simulink model "model"  (R2016a)
settings: Solver=VariableStepAuto  StartTime=0.0  StopTime=30  FixedStep=0.001  RelTol=1e-3
InitFcn:
  | InitModel;
values from neighbouring files (symbols this model uses):
  d = 100    [InitModel.m]    (also in RobotConstants.mat = 1000)
  k = 1900    [RobotConstants.mat]
  l0 = 0.16    [RobotConstants.mat]
  ls = 0.17    [RobotConstants.mat]
  m_lower = 0.5    [RobotConstants.mat]
  m_upper = 1    [RobotConstants.mat]
  n = ceil(length(q)/3)    [C.m]    (also in InitModel.m = 1; M.m; N.m; Q.m)
settings Model: Creator=Florian  LastModifiedBy=Florian
settings DataIOCC: ExternalInput=[l0]

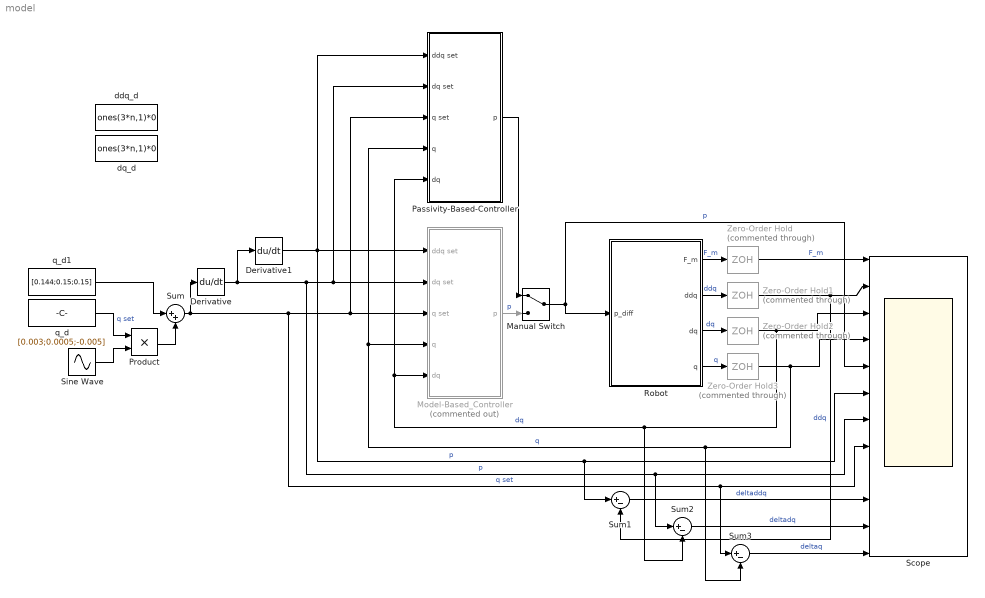
== system model ==
  Derivative : Derivative
  Derivative1 : Derivative
  Manual Switch : ManualSwitch
  Model-Based_Controller : Subsystem  Commented=on
  Passivity-Based-Controller : Subsystem
  Product : Product
  Robot : Subsystem
      mask Display: image('C:\Users\Florian\Documents\Uni\IDP\DVD\Pictures\contibot1seg.JPG');
  Scope : Scope  NumInputPorts=12
  Sine Wave : Sin  Amplitude=0.5  Bias=0.5  Phase=pi/2  SampleTime=0
  Sum : Sum  Inputs=|++
  Sum1 : Sum  Inputs=|+-
  Sum2 : Sum  Inputs=|+-
  Sum3 : Sum  Inputs=|+-
  Zero-Order Hold{,1..3} (4 alike) : ZeroOrderHold  Commented=through  SampleTime=0.01
  ddq_d : Constant  Value=ones(3*n,1)*0  SampleTime=0.01
  dq_d : Constant  Value=ones(3*n,1)*0  SampleTime=0.01
  q_d : Constant  Value=[0.003;0.0005;-0.005]  SampleTime=0.01
  q_d1 : Constant  Value=[0.144;0.15;0.15]  SampleTime=0.01
  wires:
  Robot/1(F_m) -> Zero-Order Hold/1  "F_m"
  Robot/2(ddq) -> Zero-Order Hold1/1  "ddq"
  Robot/3(dq) -> Zero-Order Hold2/1  "dq"
  Robot/4(q) -> Zero-Order Hold3/1  "q"
  Sum/1 -> Derivative/1, Sum3/1, Scope/8, Passivity-Based-Controller/3(q set), Model-Based_Controller/3(q set)  "q set"
  Zero-Order Hold/1 -> Scope/1  "F_m"
  Zero-Order Hold1/1 -> Sum1/2, Scope/2  "ddq"
  Zero-Order Hold2/1 -> Model-Based_Controller/5(dq), Passivity-Based-Controller/5(dq), Sum2/2, Scope/3  "dq"
  Zero-Order Hold3/1 -> Passivity-Based-Controller/4(q), Model-Based_Controller/4(q), Sum3/2, Scope/4  "q"
  Derivative/1 -> Passivity-Based-Controller/2(dq set), Model-Based_Controller/2(dq set), Sum2/1, Scope/7, Derivative1/1  "p"
  Derivative1/1 -> Passivity-Based-Controller/1(ddq set), Model-Based_Controller/1(ddq set), Sum1/1, Scope/6  "p"
  Manual Switch/1 -> Robot/1(p_diff), Scope/5  "p"
  Model-Based_Controller/1(p) -> Manual Switch/2  "p"
  Passivity-Based-Controller/1(p) -> Manual Switch/1
  q_d/1 -> Product/1  "q set"
  Sine Wave/1 -> Product/2
  Product/1 -> Sum/2
  q_d1/1 -> Sum/1
  Sum3/1 -> Scope/12  "deltaq"
  Sum2/1 -> Scope/11  "deltadq"
  Sum1/1 -> Scope/10  "deltaddq"

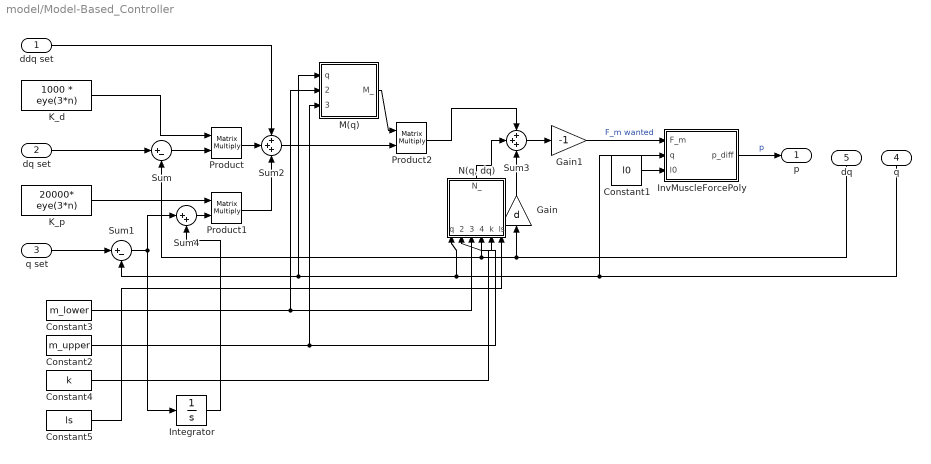
== system model/Model-Based_Controller ==
  ddq set : Inport
  dq set : Inport  Port=2
  q set : Inport  Port=3
  q : Inport  Port=4
  dq : Inport  Port=5
  Constant1 : Constant  Value=l0  SampleTime=0.01
  Constant2 : Constant  Value=m_upper
  Constant3 : Constant  Value=m_lower
  Constant4 : Constant  Value=k
  Constant5 : Constant  Value=ls
  Gain : Gain  Gain=d
  Gain1 : Gain  Gain=-1
  Integrator : Integrator  InitialCondition=zeros(3*n,1)
  InvMuscleForcePoly : MATLAB Function  TreatAsAtomicUnit=on
  K_d : Constant  Value=1000 * eye(3*n)  SampleTime=0.01
  K_p : Constant  Value=20000* eye(3*n)  SampleTime=0.01
  M(q) : MATLAB Function  TreatAsAtomicUnit=on
  "N(q, dq)" : MATLAB Function  TreatAsAtomicUnit=on
  Product : Product  Multiplication=Matrix(*)
  Product1 : Product  Multiplication=Matrix(*)
  Product2 : Product  Multiplication=Matrix(*)
  Sum : Sum  Inputs=|+-
  Sum1 : Sum  Inputs=|+-
  Sum2 : Sum  Inputs=+++
  Sum3 : Sum  Inputs=+++
  Sum4 : Sum  Inputs=|++
  p : Outport
  wires:
  Sum/1 -> Product/2
  M(q)/1(M_) -> Product2/1
  Sum2/1 -> Product2/2
  "N(q, dq)"/1(N_) -> Sum3/2
  K_p/1 -> Product1/1
  Gain/1 -> Sum3/3
  Sum1/1 -> Sum4/1, Integrator/1
  Product1/1 -> Sum2/3
  Product2/1 -> Sum3/1
  Product/1 -> Sum2/2
  Sum3/1 -> Gain1/1
  K_d/1 -> Product/1
  Constant1/1 -> InvMuscleForcePoly/3(l0)
  Gain1/1 -> InvMuscleForcePoly/1(F_m)  "F_m wanted"
  InvMuscleForcePoly/1(p_diff) -> p/1  "p"
  dq/1 -> Sum/2, "N(q, dq)"/2(dq), Gain/1
  q set/1 -> Sum1/1
  q/1 -> Sum1/2, M(q)/1(q), "N(q, dq)"/1(q), InvMuscleForcePoly/2(q)
  dq set/1 -> Sum/1
  ddq set/1 -> Sum2/1
  Constant3/1 -> M(q)/2(m_lower), "N(q, dq)"/3(m_lower)
  Constant2/1 -> M(q)/3(m_upper), "N(q, dq)"/4(m_upper)
  Constant4/1 -> "N(q, dq)"/5(k)
  Constant5/1 -> "N(q, dq)"/6(ls)
  Integrator/1 -> Sum4/2
  Sum4/1 -> Product1/2

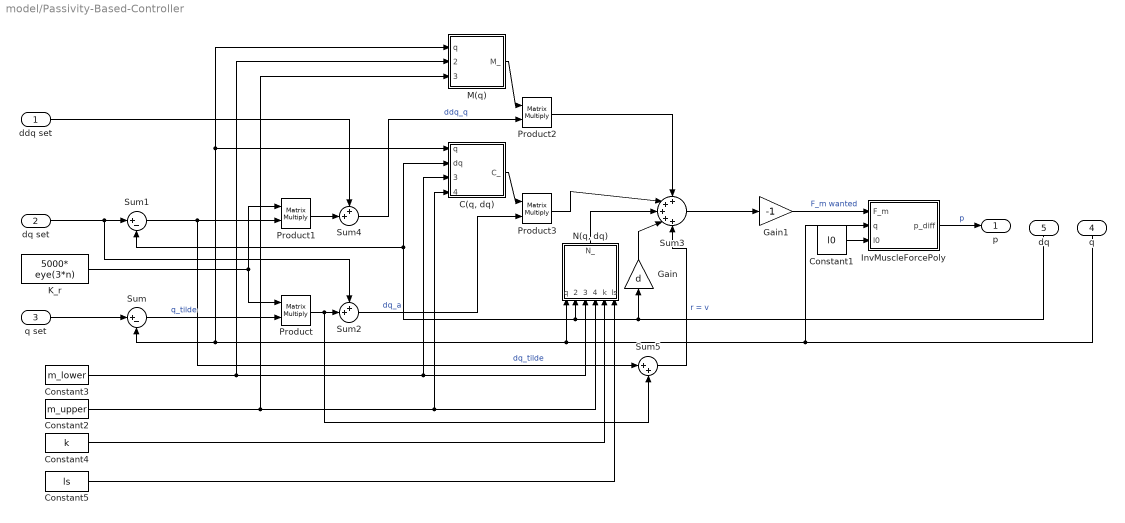
== system model/Passivity-Based-Controller ==
  ddq set : Inport
  dq set : Inport  Port=2
  q set : Inport  Port=3
  q : Inport  Port=4
  dq : Inport  Port=5
  "C(q, dq)" : MATLAB Function  TreatAsAtomicUnit=on
  Constant1 : Constant  Value=l0  SampleTime=0.01
  Constant2 : Constant  Value=m_upper
  Constant3 : Constant  Value=m_lower
  Constant4 : Constant  Value=k
  Constant5 : Constant  Value=ls
  Gain : Gain  Gain=d
  Gain1 : Gain  Gain=-1
  InvMuscleForcePoly : MATLAB Function  TreatAsAtomicUnit=on
  K_r : Constant  Value=5000* eye(3*n)  SampleTime=0.01
  M(q) : MATLAB Function  TreatAsAtomicUnit=on
  "N(q, dq)" : MATLAB Function  TreatAsAtomicUnit=on
  Product{,1..3} (4 alike) : Product  Multiplication=Matrix(*)
  Sum : Sum  Inputs=|+-
  Sum1 : Sum  Inputs=|+-
  Sum2 : Sum  Inputs=++|
  Sum3 : Sum  Inputs=+++++
  Sum4 : Sum  Inputs=++|
  Sum5 : Sum  Inputs=|++
  p : Outport
  wires:
  M(q)/1(M_) -> Product2/1
  "N(q, dq)"/1(N_) -> Sum3/3
  Gain/1 -> Sum3/4
  Product2/1 -> Sum3/1
  Sum3/1 -> Gain1/1
  Constant1/1 -> InvMuscleForcePoly/3(l0)
  Gain1/1 -> InvMuscleForcePoly/1(F_m)  "F_m wanted"
  InvMuscleForcePoly/1(p_diff) -> p/1  "p"
  dq/1 -> "C(q, dq)"/2(dq), Sum1/2, "N(q, dq)"/2(dq), Gain/1
  q/1 -> "N(q, dq)"/1(q), "C(q, dq)"/1(q), M(q)/1(q), Sum/2, InvMuscleForcePoly/2(q)
  q set/1 -> Sum/1
  Sum/1 -> Product/2  "q_tilde"
  dq set/1 -> Sum2/1, Sum1/1
  Constant3/1 -> "C(q, dq)"/3(m_lower), "N(q, dq)"/3(m_lower), M(q)/2(m_lower)
  Constant2/1 -> "C(q, dq)"/4(m_upper), "N(q, dq)"/4(m_upper), M(q)/3(m_upper)
  Constant4/1 -> "N(q, dq)"/5(k)
  Constant5/1 -> "N(q, dq)"/6(ls)
  Sum1/1 -> Sum5/1, Product1/2  "dq_tilde"
  K_r/1 -> Product1/1, Product/1
  Product/1 -> Sum5/2, Sum2/2
  Product1/1 -> Sum4/2
  ddq set/1 -> Sum4/1
  Sum4/1 -> Product2/2  "ddq_q"
  Sum2/1 -> Product3/2  "dq_a"
  "C(q, dq)"/1(C_) -> Product3/1
  Product3/1 -> Sum3/2
  Sum5/1 -> Sum3/5  "r = v"

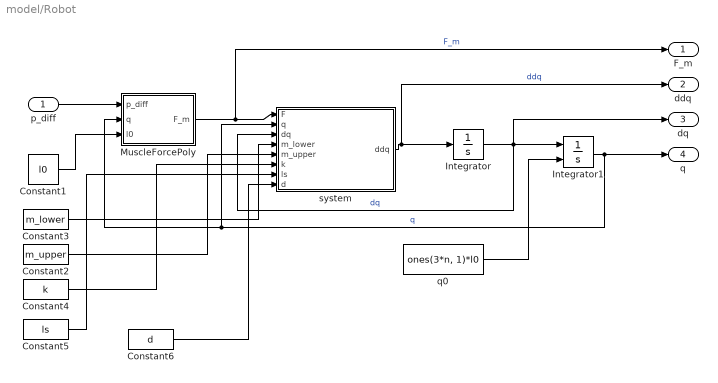
== system model/Robot ==
  p_diff : Inport
  Constant1 : Constant  Value=l0
  Constant2 : Constant  Value=m_upper
  Constant3 : Constant  Value=m_lower
  Constant4 : Constant  Value=k
  Constant5 : Constant  Value=ls
  Constant6 : Constant  Value=d
  Integrator : Integrator  InitialCondition=ones(3*n, 1)*0
  Integrator1 : Integrator  InitialConditionSource=external  InitialCondition=[0.17; 0.15; 0.15]
  MuscleForcePoly : MATLAB Function  TreatAsAtomicUnit=on
  q0 : Constant  Value=ones(3*n, 1)*l0
  system : MATLAB Function  TreatAsAtomicUnit=on
  F_m : Outport
  ddq : Outport  Port=2
  dq : Outport  Port=3
  q : Outport  Port=4
  wires:
  MuscleForcePoly/1(F_m) -> system/1(F), F_m/1  "F_m"
  q0/1 -> Integrator1/2
  system/1(ddq) -> ddq/1, Integrator/1  "ddq"
  Integrator1/1 -> q/1, MuscleForcePoly/2(q), system/2(q)  "q"
  Integrator/1 -> dq/1, system/3(dq), Integrator1/1  "dq"
  p_diff/1 -> MuscleForcePoly/1(p_diff)
  Constant1/1 -> MuscleForcePoly/3(l0)
  Constant3/1 -> system/4(m_lower)
  Constant2/1 -> system/5(m_upper)
  Constant4/1 -> system/6(k)
  Constant5/1 -> system/7(ls)
  Constant6/1 -> system/8(d)

== matlab function model/Robot/MuscleForcePoly ==
  data: p_diff input; F_m output; q input; l0 input
function F_m = fcn(p_diff, q, l0)
%#codegen

%coder.extrinsic('Ffunc');

a1 =         142;
b1 =     0.09406;
c1 =       1.282;
a2 =       106.3;
b2 =      0.1212;
c2 =      -1.436;
a3 =       4.354;
b3 =       0.401;
c3 =     -0.8088;
a4 =        1.19;
b4 =      0.7829;
c4 =      -2.241;
a5 =       2.532;
b5 =      0.5635;
c5 =      -1.872;
a6 =        1.02;
b6 =      0.9889;
c6 =      -2.835;

F_m = a1*sin(b1*p_diff+c1) + a2*sin(b2*p_diff+c2) + a3*sin(b3*p_diff+c3) + ...
      a4*sin(b4*p_diff+c4) + a5*sin(b5*p_diff+c5) + a6*sin(b6*p_diff+c6);

== matlab function model/Robot/system ==
  data: F input; ddq output; q input; dq input; m_lower input; m_upper input; k input; ls input; d input
function ddq = fcn(F, q, dq, m_lower, m_upper, k, ls, d)
%#codegen

%coder.extrinsic('M');
%coder.extrinsic('N');

M_ = zeros(length(q));
C_ = zeros(length(q));
N_ = zeros(length(q), 1);

for i = 1:floor(length(q)/3)
    if abs(q(i*3-2) - q(i*3-1)) < 0.0001 && abs(q(i*3-1) - q(i*3)) < 0.0001
        q(i*3-2) = q(i*3-2) + 0.0001;
    end
end

M_ = M(q, m_lower, m_upper);
C_ = C(q, dq, m_lower, m_upper);
N_ = -N(q, m_lower, m_upper, k, ls);  
 
Q_ = Q(-F, q, dq, d);  


invM = pinv(M_);
ddq = invM * (Q_ - N_ - C_*dq);

== matlab function model/Model-Based_Controller/M(q) ==
  data: M_ output; q input; m_lower input; m_upper input
function M_ = fcn(q, m_lower, m_upper)
%#codegen

for i = 1:floor(length(q)/3)
    if abs(q(i*3-2) - q(i*3-1)) < 0.0001 && abs(q(i*3-1) - q(i*3)) < 0.0001
        q(i*3-2) = q(i*3-2) + 0.0001;
    end
end

M_ = M(q, m_lower, m_upper);

== matlab function model/Model-Based_Controller/N(q, dq) ==
  data: N_ output; q input; dq input; m_lower input; m_upper input; k input; ls input
function N_ = fcn(q, dq, m_lower, m_upper, k, ls)
%#codegen

for i = 1:floor(length(q)/3)
    if abs(q(i*3-2) - q(i*3-1)) < 0.0001 && abs(q(i*3-1) - q(i*3)) < 0.0001
        q(i*3-2) = q(i*3-2) + 0.0001;
    end
end

N_ = -N(q, m_lower, m_upper, k, ls);

== matlab function model/Model-Based_Controller/InvMuscleForcePoly ==
  data: F_m input; p_diff output; q input; l0 input
function p_diff = fcn(F_m, q, l0)
%#codegen

p1 =   7.551e-05;
p2 =    -0.01115;
p3 =      0.6236;
p4 =      -9.759;

p_diff = p1*F_m.^3 + p2*F_m.^2 + p3*F_m + p4;

for i = 1:length(p_diff)
    if p_diff(i) < 0
        p_diff(i) = 0;
    elseif p_diff(i) > 6
        p_diff(i) = 6;
    end
end

== matlab function model/Passivity-Based-Controller/InvMuscleForcePoly ==
  data: F_m input; p_diff output; q input; l0 input
function p_diff = fcn(F_m, q, l0)
%#codegen

p1 =   7.551e-05;
p2 =    -0.01115;
p3 =      0.6236;
p4 =      -9.759;

p_diff = p1*F_m.^3 + p2*F_m.^2 + p3*F_m + p4;

for i = 1:length(p_diff)
    if p_diff(i) < 0
        p_diff(i) = 0;
    elseif p_diff(i) > 6
        p_diff(i) = 6;
    end
end

== matlab function model/Passivity-Based-Controller/M(q) ==
  data: M_ output; q input; m_lower input; m_upper input
function M_ = fcn(q, m_lower, m_upper)
%#codegen

for i = 1:floor(length(q)/3)
    if abs(q(i*3-2) - q(i*3-1)) < 0.0001 && abs(q(i*3-1) - q(i*3)) < 0.0001
        q(i*3-2) = q(i*3-2) + 0.0001;
    end
end

M_ = M(q, m_lower, m_upper);

== matlab function model/Passivity-Based-Controller/N(q, dq) ==
  data: N_ output; q input; dq input; m_lower input; m_upper input; k input; ls input
function N_ = fcn(q, dq, m_lower, m_upper, k, ls)
%#codegen

for i = 1:floor(length(q)/3)
    if abs(q(i*3-2) - q(i*3-1)) < 0.0001 && abs(q(i*3-1) - q(i*3)) < 0.0001
        q(i*3-2) = q(i*3-2) + 0.0001;
    end
end

N_ = -N(q, m_lower, m_upper, k, ls);

== matlab function model/Passivity-Based-Controller/C(q, dq) ==
  data: C_ output; q input; dq input; m_lower input; m_upper input
function C_ = fcn(q, dq, m_lower, m_upper)
%#codegen

for i = 1:floor(length(q)/3)
    if abs(q(i*3-2) - q(i*3-1)) < 0.0001 && abs(q(i*3-1) - q(i*3)) < 0.0001
        q(i*3-2) = q(i*3-2) + 0.0001;
    end
end

C_ = C(q, dq, m_lower, m_upper);
